simulink model "section4_6"  (R2020a)
settings: Solver=VariableStepAuto  StartTime=0.0  StopTime=2.8  RelTol=1e-3
values from neighbouring files (symbols this model uses):
  K = 6.85/4    (= 1.7125)    [simulatePIDResponse.m]    (also in stepResponseTesting.m = 2.74)
  sigma = 10    [simulatePIDResponse.m]    (also in stepResponseTesting.m)
settings Model: Creator=broom  LastModifiedBy=broom

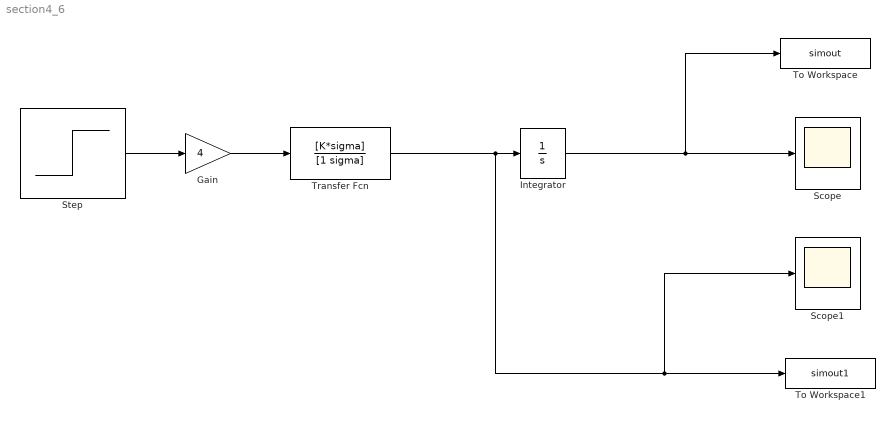
== system section4_6 ==
  Gain : Gain  Gain=4
  Integrator : Integrator
  Scope : Scope
  Scope1 : Scope
  Step : Step  SampleTime=0
  To Workspace : ToWorkspace  VariableName=simout  SaveFormat=Timeseries  SampleTime=-1
  To Workspace1 : ToWorkspace  VariableName=simout1  SaveFormat=Timeseries  SampleTime=-1
  Transfer Fcn : TransferFcn  Numerator=[K*sigma]  Denominator=[1 sigma]
  wires:
  Integrator/1 -> To Workspace/1, Scope/1
  Transfer Fcn/1 -> Scope1/1, To Workspace1/1, Integrator/1
  Step/1 -> Gain/1
  Gain/1 -> Transfer Fcn/1
